simulink model "TV_comparison"  (R2022a)
settings: Solver=VariableStepAuto  StartTime=0.0  StopTime=140  RelTol=1e-3
values from neighbouring files (symbols this model uses):
  Battery_Voltage = 120    [RCVD.mat]
  CG_height = 0.6    [RCVD.mat]
  Cornering_Stiffness = 1000    [RCVD.mat]
  Gear_ratio = 6    [RCVD.mat]
  Mass = 250    [RCVD.mat]
  track_cumulative = tc.track_cumulative    [mlx_is_terrible.m]    (also in track.mat = [-1 0 1 0 0 -1 1 0 -1 1 -1 1 ... (560 elements, 140x4)])
  Wheel_Base = 1.8    [RCVD.mat]
  Wheel_Radius = 0.211    [RCVD.mat]
  Width = 1    [RCVD.mat]
libraries: SignalEditorBlockLib x4, autolibmappedmotor x2
settings Model: Creator=gautamd  LastModifiedBy=gautamd

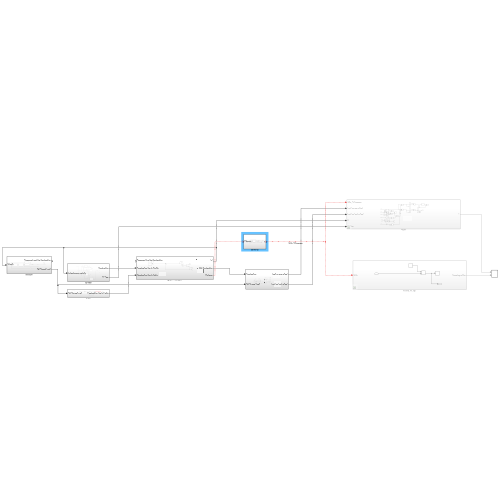
[thumbnail: Simulink's stored preview of the top-level diagram]
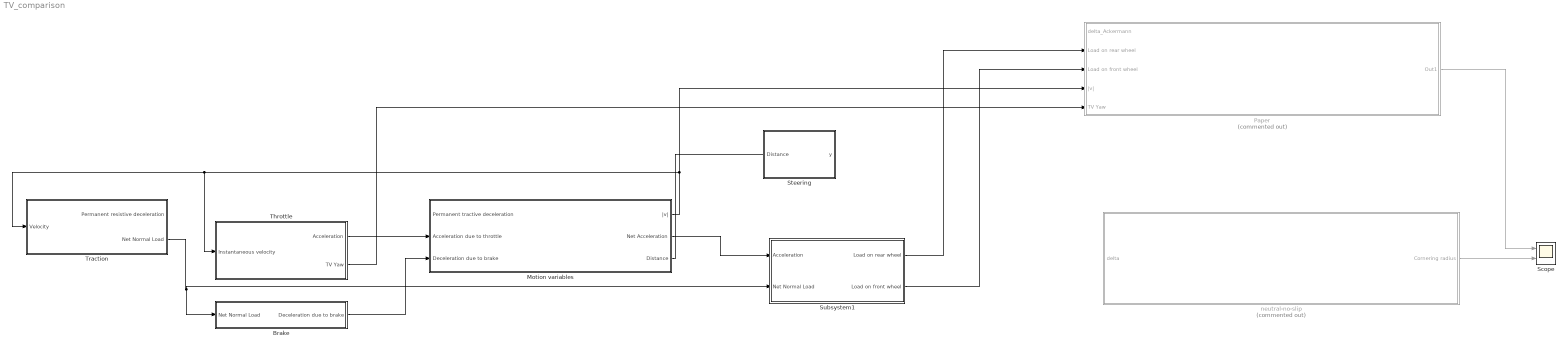
== system TV_comparison ==
  Brake : Subsystem
  Motion variables : Subsystem
  Paper : Subsystem  Commented=on
  Scope : Scope  NumInputPorts=2
  Steering : Subsystem
  Subsystem1 : Subsystem
  Throttle : Subsystem
  Traction : Subsystem
  neutral-no-slip : Subsystem  Commented=on
  wires:
  ? -> neutral-no-slip/1(delta), Paper/1(delta_Ackermann)  "delta_Ackermann"
  Subsystem1/1(Load on rear wheel) -> Paper/2(Load on rear wheel)
  Motion variables/2(Net Acceleration) -> Subsystem1/1(Acceleration)
  Subsystem1/2(Load on front wheel) -> Paper/3(Load on front wheel)
  Throttle/2(TV Yaw) -> Paper/5(TV Yaw)
  neutral-no-slip/1(Cornering radius) -> Scope/2
  Motion variables/1(|v|) -> Traction/1(Velocity), Throttle/1(Instantaneous velocity), Paper/4(|v|)
  Throttle/1(Acceleration) -> Motion variables/2(Acceleration due to throttle)
  Traction/2(Net Normal Load) -> Brake/1(Net Normal Load), Subsystem1/2(Net Normal Load)
  Paper/1(Out1) -> Scope/1
  Brake/1(Deceleration due to brake) -> Motion variables/3(Deceleration due to brake)
  Motion variables/3(Distance) -> ?

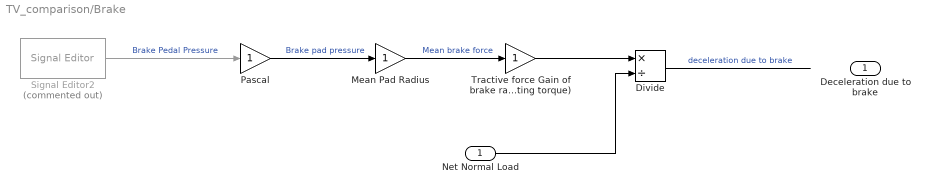
== system TV_comparison/Brake ==
  Net Normal Load : Inport
  Divide : Product  Inputs=*/
  Mean Pad Radius : Gain
  Pascal : Gain
  Signal Editor2 : SignalEditorBlockLib/Signal Editor  Commented=on  FileName=Brake_map.mat  ActiveScenario=Scenario  ActiveSignal=Signal 1  IsBus=off  OutputBusObjectStr=Bus: BusObject  SampleTime=0  Interpolate=off  ZeroCross=off  OutputAfterFinalValue=Setting to zero  Unit=inherit  PreserveSignalName=on
  Tractive force Gain of brake radius / wheel radius (equating torque) : Gain
  Deceleration due to brake : Outport
  wires:
  Signal Editor2/1 -> Pascal/1  "Brake Pedal Pressure"
  Pascal/1 -> Mean Pad Radius/1  "Brake pad pressure"
  Mean Pad Radius/1 -> Tractive force Gain of brake radius / wheel radius (equating torque)/1  "Mean brake force"
  Tractive force Gain of brake radius / wheel radius (equating torque)/1 -> Divide/1
  Divide/1 -> ?  "deceleration due to brake"
  Net Normal Load/1 -> Divide/2

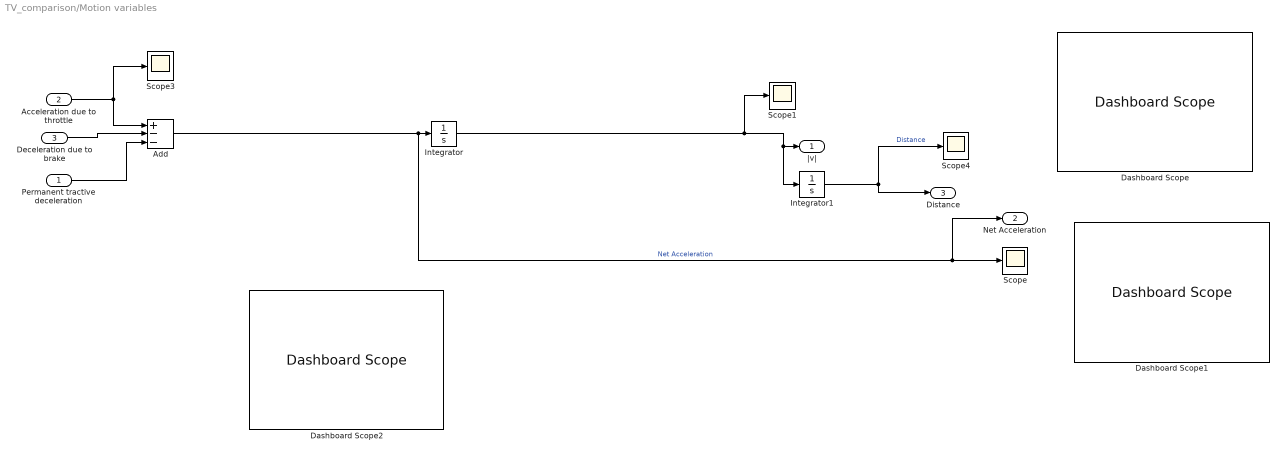
== system TV_comparison/Motion variables ==
  Permanent tractive deceleration : Inport
  Acceleration due to throttle : Inport  Port=2
  Deceleration due to brake : Inport  Port=3
  Add : Sum  Inputs=+--
  Dashboard Scope : DashboardScope
  Dashboard Scope1 : DashboardScope
  Dashboard Scope2 : DashboardScope
  Integrator : Integrator
  Integrator1 : Integrator
  Scope{,1,3..4} (4 alike) : Scope
  |v| : Outport
  Net Acceleration : Outport  Port=2
  Distance : Outport  Port=3
  wires:
  Integrator1/1 -> Scope4/1, Distance/1  "Distance"
  Add/1 -> Net Acceleration/1, Scope/1, Integrator/1  "Net Acceleration"
  Permanent tractive deceleration/1 -> Add/3
  Acceleration due to throttle/1 -> Add/1, Scope3/1
  Deceleration due to brake/1 -> Add/2
  Integrator/1 -> Scope1/1, Integrator1/1, |v|/1

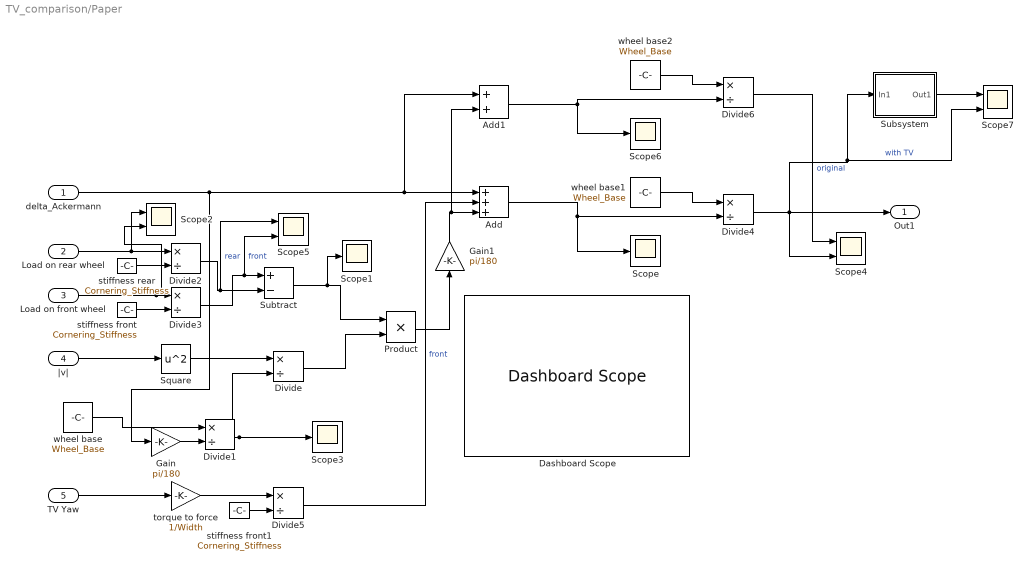
== system TV_comparison/Paper ==
  delta_Ackermann : Inport
  Load on rear wheel : Inport  Port=2
  Load on front wheel : Inport  Port=3
  |v| : Inport  Port=4
  TV Yaw : Inport  Port=5
  Add : Sum  Inputs=+++
  Add1 : Sum
  Dashboard Scope : DashboardScope
  Divide{,1..6} (7 alike) : Product  Inputs=*/
  Gain : Gain  Gain=pi/180
  Gain1 : Gain  Gain=pi/180
  Product : Product
  Scope{,1,3,6} (4 alike) : Scope
  Scope{2,4..5,7} (4 alike) : Scope  NumInputPorts=2
  Square : Math  Operator=square
  Subsystem : Subsystem
  Subtract : Sum  Inputs=+-
  stiffness front : Constant  Value=Cornering_Stiffness
  stiffness front1 : Constant  Value=Cornering_Stiffness
  stiffness rear : Constant  Value=Cornering_Stiffness
  torque to force : Gain  Gain=1/Width
  wheel base : Constant  Value=Wheel_Base
  wheel base1 : Constant  Value=Wheel_Base
  wheel base2 : Constant  Value=Wheel_Base
  Out1 : Outport
  wires:
  delta_Ackermann/1 -> Gain/1, Add1/1, Add/1
  |v|/1 -> Square/1
  Square/1 -> Divide/1
  wheel base/1 -> Divide1/1
  Divide1/1 -> Divide/2, Scope3/1
  Load on rear wheel/1 -> Scope2/1, Divide2/1
  Load on front wheel/1 -> Scope2/2, Divide3/1
  stiffness rear/1 -> Divide2/2
  stiffness front/1 -> Divide3/2
  Divide3/1 -> Scope5/2, Subtract/1  "front"
  Divide2/1 -> Subtract/2, Scope5/1  "rear"
  Subtract/1 -> Scope1/1, Product/1
  Divide/1 -> Product/2
  Product/1 -> Gain1/1
  Add/1 -> Divide4/2, Scope/1
  Gain/1 -> Divide1/2
  Divide4/1 -> Scope7/2, Subsystem/1(In1), Scope4/2, Out1/1  "with TV"
  wheel base1/1 -> Divide4/1
  Gain1/1 -> Add1/2, Add/3
  TV Yaw/1 -> torque to force/1
  torque to force/1 -> Divide5/1
  stiffness front1/1 -> Divide5/2
  Divide5/1 -> Add/2  "front"
  wheel base2/1 -> Divide6/1
  Add1/1 -> Divide6/2, Scope6/1
  Divide6/1 -> Scope4/1  "original"
  Subsystem/1(Out1) -> Scope7/1

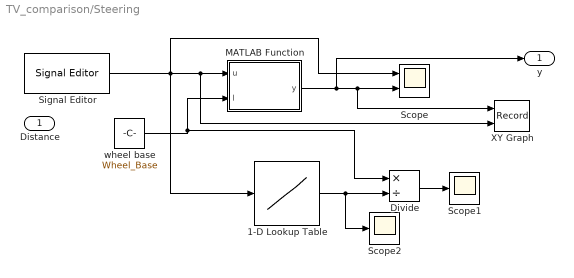
== system TV_comparison/Steering ==
  Distance : Inport
  1-D Lookup Table : Lookup_n-D  NumberOfTableDimensions=1  BreakpointsForDimension1=track_cumulative(:,4,:) - track_cumulative(:,2,:)  Table=track_cumulative(:,3,:).*track_cumulative(:,1,:)  InterpMethod=Flat  InternalRulePriority=Speed  RndMeth=Simplest
  Divide : Product  Inputs=*/
  MATLAB Function : MATLAB Function  TreatAsAtomicUnit=on
  Scope : Scope  NumInputPorts=2
  Scope1 : Scope
  Scope2 : Scope
  Signal Editor : SignalEditorBlockLib/Signal Editor  FileName=temp_distance_vs_time.mat  ActiveScenario=Scenario  ActiveSignal=Signal 1  IsBus=off  OutputBusObjectStr=Bus: BusObject  SampleTime=0  ZeroCross=off  OutputAfterFinalValue=Setting to zero  Unit=inherit  PreserveSignalName=on
  XY Graph : Record  FileSettingsInternal="{\"entries\":[{\"content\":{\"excelSettings\":{\"content\":{},\"type\":\"Streamout.ExcelSettings\"}},\"type\":\"Streamout.FileSettingStorage\",\"uuid\":\"\"}],\"packageUris\":[\"http:\\/\\/schema.mathworks.com\\/mf0\\/streamout_blocks\\/R2020a\"],\"version\":\"1.0\"}"  Layout=[1 1]  SignalsInternal="{\"entries\":[{\"content\":{\"signals\":[{\"content\":{\"blockPath\":[],\"channel\":[],\"dimensions\":[1],\"domain\":\"\",\"lineColor\":\"#a2142f\",\"plots\":[],\"port\":1,\"sid\":[\"\"],\"signalID\":2948,\"signalName\":\"MATLAB Function\"},\"type\":\"RecordBlkView.Signal\",\"uuid\":\"\"},{\"content\":{\"blockPath\":[],\"channel\":[],\"dimensions\":[1],\"domain\":\"\",\"lineColor\":\"#139fff\",\"plots\":[],\"port\":2,\"sid\":[\"\"],\"signalID\":2952,\"signalName\":\"Signal Editor\"},\"type\":\"RecordBlkView.Signal\",\"uuid\":\"\"}]},\"type\":\"RecordBlkView.InputSignals\",\"uuid\":\"\"}],\"packageUris\":[\"http:\\/\\/schema.mathworks.com\\/mf0\\/streamout_blocks\\/R2020a\"],\"version\":\"1.0\"}"  VisualizationBindings="{\"xyplotplugin\":{\"info\":[{\"series\":[],\"subplotID\":1}]}}"  CompatibilityTag=XY
  wheel base : Constant  Value=Wheel_Base
  y : Outport
  wires:
  Signal Editor/1 -> 1-D Lookup Table/1, Scope/1, XY Graph/2, MATLAB Function/1(u)
  wheel base/1 -> Divide/1, MATLAB Function/2(l)
  MATLAB Function/1(y) -> y/1, XY Graph/1, Scope/2
  1-D Lookup Table/1 -> Scope2/1, Divide/2
  Divide/1 -> Scope1/1

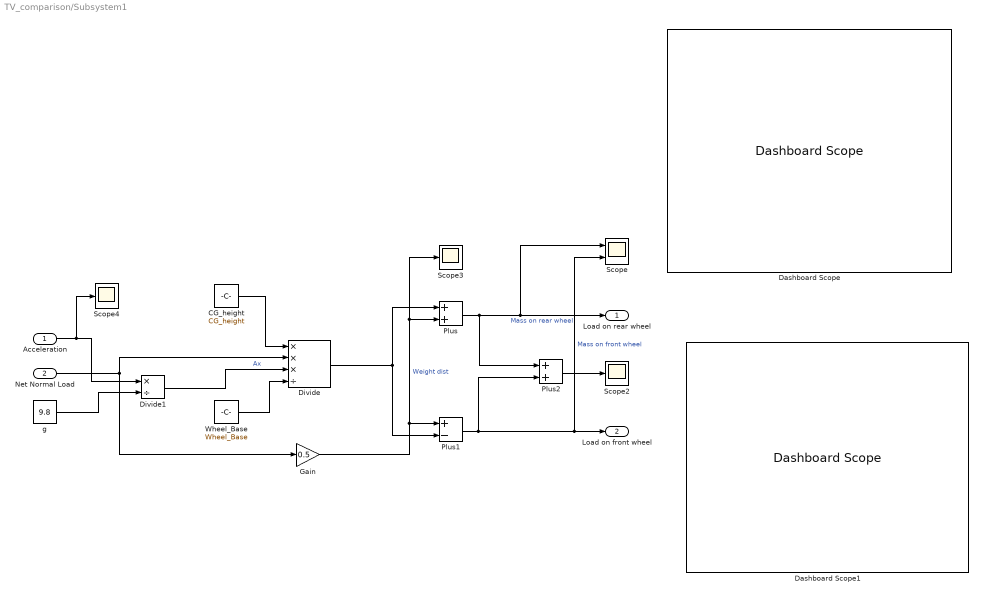
== system TV_comparison/Subsystem1 ==
  Acceleration : Inport
  Net Normal Load : Inport  Port=2
  CG_height : Constant  Value=CG_height
  Dashboard Scope : DashboardScope
  Dashboard Scope1 : DashboardScope
  Divide : Product  Inputs=***/
  Divide1 : Product  Inputs=*/
  Gain : Gain  Gain=0.5
  Plus : Sum
  Plus1 : Sum  Inputs=+-
  Plus2 : Sum
  Scope : Scope  NumInputPorts=2
  Scope2 : Scope
  Scope3 : Scope
  Scope4 : Scope
  Wheel_Base : Constant  Value=Wheel_Base
  g : Constant  Value=9.8
  Load on rear wheel : Outport
  Load on front wheel : Outport  Port=2
  wires:
  g/1 -> Divide1/2
  Divide/1 -> Plus1/2, Plus/1
  Acceleration/1 -> Scope4/1, Divide1/1
  Gain/1 -> Scope3/1, Plus/2, Plus1/1  "Weight dist"
  CG_height/1 -> Divide/1
  Wheel_Base/1 -> Divide/4
  Divide1/1 -> Divide/3  "Ax"
  Plus/1 -> Scope/1, Load on rear wheel/1, Plus2/1  "Mass on rear wheel"
  Plus1/1 -> Scope/2, Load on front wheel/1, Plus2/2  "Mass on front wheel"
  Net Normal Load/1 -> Divide/2, Gain/1
  Plus2/1 -> Scope2/1

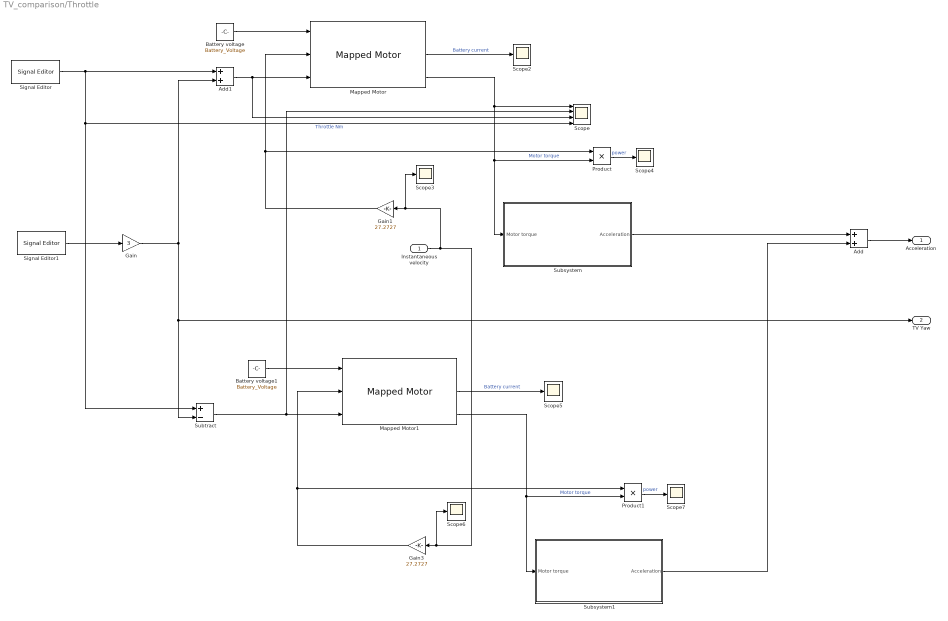
== system TV_comparison/Throttle ==
  Instantaneous velocity : Inport
  Add : Sum
  Add1 : Sum
  Battery voltage : Constant  Value=Battery_Voltage
  Battery voltage1 : Constant  Value=Battery_Voltage
  Gain : Gain  Gain=3
  Gain1 : Gain  Gain=27.2727
  Gain3 : Gain  Gain=27.2727
  Mapped Motor : autolibmappedmotor/Mapped Motor  port_config=Speed  param_by=Maximum torque and power  w_t=[ 0 375 750 800 ]  T_t=[0.09 0.08 0.07 0]  torque_max=29  power_max=Max_Power  Tc=0.1  param_loss=Single efficiency measurement  eff=93  w_eff=600  T_eff=29  Piron=0  Pbase=0  w_eff_bp=[-8000 -4000 0 4000 8000]  T_eff_bp=[0 0.03 0.06 0.09]  Temp_eff_bp=[233.15 293.15 373.15]  losses_table=[1.49 1.67 2.21 3.10; 0.42 0.69 1.14 2.03; 0.06 0.24 0.78 1.68; 0.42 0.69 1.14 2.03; 1.49 1.67 2.21 3.10]  losses_table_3d=cat(3,1.05*[1.49 1.67 2.21 3.10; 0.42 0.69 1.14 2.03; 0.06 0.24 0.78 1.68; 0.42 0.69 1.14 2.03; 1.49 1.67 2.21 3.10],[1.49 1.67 2.21 3.10; 0.42 0.69 1.14 2.03; 0.06 0.24 0.78 1.68; 0.42 0.69 1.14 2.03; 1.49 1.67 2.21 3.10],1.03*[1.49 1.67 2.21 3.10; 0.42 0.69 1.14 2.03; 0.06 0.24 0.78 1.68; 0.42 0.69 1.14 2.03; 1.49 1.67 2.21 3.10])  efficiency_table=[95 95 95 95; 95 95 95 95; 95 95 95 95; 95 95 95 95; 95 95 95 95]  efficiency_table_3d=cat(3,90*ones(5,4),95*ones(5,4),92*ones(5,4))  J=0.021  b=1e-5  omega_o=0  T_t_extended=[0 0.07 0.08 0.09 0.08 0.07 0]  w_t_extended=[-800 -750 -375 0 375 750 800]  KLossIron=0  KLossCopper=1.5573  x_w_eff_vec=[-8000 -4000 0 4000 8000]  x_T_eff_vec=[-0.09 -0.06 -0.03 0 0.03 0.06 0.09]  x_tmp_eff_vec=[233.15 293.15 373.15]  x_losses_mat=[3.1 2.21 1.67 1.49 1.67 2.21 3.1;2.03 1.14 0.69 0.42 0.69 1.14 2.03;1.68 0.78 0.24 0.06 0.24 0.78 1.68;2.03 1.14 0.69 0.42 0.69 1.14 2.03;3.1 2.21 1.67 1.49 1.67 2.21 3.1]  x_losses_mat_3d=cat(3,[3.255 2.3205 1.7535 1.5645 1.7535 2.3205 3.255;2.1315 1.197 0.7245 0.441 0.7245 1.197 2.1315;1.764 0.819 0.252 0.063 0.252 0.819 1.764;2.1315 1.197 0.7245 0.441 0.7245 1.197 2.1315;3.255 2.3205 1.7535 1.5645 1.7535 2.3205 3.255],[3.1 2.21 1.67 1.49 1.67 2.21 3.1;2.03 1.14 0.69 0.42 0.69 1.14 2.03;1.68 0.78 0.24 0.06 0.24 0.78 1.68;2.03 1.14 0.69 0.42 0.69 1.14 2.03;3.1 2.21 1.67 1.49 1.67 2.21 3.1],[3.193 2.2763 1.7201 1.5347 1.7201 2.2763 3.193;2.0909 1.1742 0.7107 0.4326 0.7107 1.1742 2.0909;1.7304 0.8034 0.2472 0.0618 0.2472 0.8034 1.7304;2.0909 1.1742 0.7107 0.4326 0.7107 1.1742 2.0909;3.193 2.2763 1.7201 1.5347 1.7201 2.2763 3.193])  CalLossMapData={}  CalLossWithTempMapData={}  aMode=2  RefBlkName='autolibmappedmotor/Mapped Motor'
      settings: SourceProductBaseCode=PW,DR,MT,VE
  Mapped Motor1 : autolibmappedmotor/Mapped Motor  port_config=Speed  param_by=Maximum torque and power  w_t=[ 0 375 750 800 ]  T_t=[0.09 0.08 0.07 0]  torque_max=29  power_max=Max_Power  Tc=0.1  param_loss=Single efficiency measurement  eff=93  w_eff=600  T_eff=29  Piron=0  Pbase=0  w_eff_bp=[-8000 -4000 0 4000 8000]  T_eff_bp=[0 0.03 0.06 0.09]  Temp_eff_bp=[233.15 293.15 373.15]  losses_table=[1.49 1.67 2.21 3.10; 0.42 0.69 1.14 2.03; 0.06 0.24 0.78 1.68; 0.42 0.69 1.14 2.03; 1.49 1.67 2.21 3.10]  losses_table_3d=cat(3,1.05*[1.49 1.67 2.21 3.10; 0.42 0.69 1.14 2.03; 0.06 0.24 0.78 1.68; 0.42 0.69 1.14 2.03; 1.49 1.67 2.21 3.10],[1.49 1.67 2.21 3.10; 0.42 0.69 1.14 2.03; 0.06 0.24 0.78 1.68; 0.42 0.69 1.14 2.03; 1.49 1.67 2.21 3.10],1.03*[1.49 1.67 2.21 3.10; 0.42 0.69 1.14 2.03; 0.06 0.24 0.78 1.68; 0.42 0.69 1.14 2.03; 1.49 1.67 2.21 3.10])  efficiency_table=[95 95 95 95; 95 95 95 95; 95 95 95 95; 95 95 95 95; 95 95 95 95]  efficiency_table_3d=cat(3,90*ones(5,4),95*ones(5,4),92*ones(5,4))  J=0.021  b=1e-5  omega_o=0  T_t_extended=[0 0.07 0.08 0.09 0.08 0.07 0]  w_t_extended=[-800 -750 -375 0 375 750 800]  KLossIron=0  KLossCopper=1.5573  x_w_eff_vec=[-8000 -4000 0 4000 8000]  x_T_eff_vec=[-0.09 -0.06 -0.03 0 0.03 0.06 0.09]  x_tmp_eff_vec=[233.15 293.15 373.15]  x_losses_mat=[3.1 2.21 1.67 1.49 1.67 2.21 3.1;2.03 1.14 0.69 0.42 0.69 1.14 2.03;1.68 0.78 0.24 0.06 0.24 0.78 1.68;2.03 1.14 0.69 0.42 0.69 1.14 2.03;3.1 2.21 1.67 1.49 1.67 2.21 3.1]  x_losses_mat_3d=cat(3,[3.255 2.3205 1.7535 1.5645 1.7535 2.3205 3.255;2.1315 1.197 0.7245 0.441 0.7245 1.197 2.1315;1.764 0.819 0.252 0.063 0.252 0.819 1.764;2.1315 1.197 0.7245 0.441 0.7245 1.197 2.1315;3.255 2.3205 1.7535 1.5645 1.7535 2.3205 3.255],[3.1 2.21 1.67 1.49 1.67 2.21 3.1;2.03 1.14 0.69 0.42 0.69 1.14 2.03;1.68 0.78 0.24 0.06 0.24 0.78 1.68;2.03 1.14 0.69 0.42 0.69 1.14 2.03;3.1 2.21 1.67 1.49 1.67 2.21 3.1],[3.193 2.2763 1.7201 1.5347 1.7201 2.2763 3.193;2.0909 1.1742 0.7107 0.4326 0.7107 1.1742 2.0909;1.7304 0.8034 0.2472 0.0618 0.2472 0.8034 1.7304;2.0909 1.1742 0.7107 0.4326 0.7107 1.1742 2.0909;3.193 2.2763 1.7201 1.5347 1.7201 2.2763 3.193])  CalLossMapData={}  CalLossWithTempMapData={}  aMode=2  RefBlkName='autolibmappedmotor/Mapped Motor'
      settings: SourceProductBaseCode=PW,DR,MT,VE
  Product : Product
  Product1 : Product
  Scope : Scope  NumInputPorts=4
  Scope{2..7} (6 alike) : Scope
  Signal Editor : SignalEditorBlockLib/Signal Editor  FileName=Throttle_map.mat  ActiveScenario=Scenario  ActiveSignal=Signal 1  IsBus=off  OutputBusObjectStr=Bus: BusObject  SampleTime=0  Interpolate=off  ZeroCross=off  OutputAfterFinalValue=Setting to zero  Unit=inherit  PreserveSignalName=on
  Signal Editor1 : SignalEditorBlockLib/Signal Editor  FileName=Torque vectoring input.mat  ActiveScenario=Scenario  ActiveSignal=Signal 1  IsBus=off  OutputBusObjectStr=Bus: BusObject  SampleTime=0  Interpolate=off  ZeroCross=off  OutputAfterFinalValue=Setting to zero  Unit=inherit  PreserveSignalName=on
  Subsystem : Subsystem
  Subsystem1 : Subsystem
  Subtract : Sum  Inputs=+-
  Acceleration : Outport
  TV Yaw : Outport  Port=2
  wires:
  Battery voltage/1 -> Mapped Motor/1
  Signal Editor/1 -> Scope/4, Subtract/1, Add1/1  "Throttle Nm"
  Mapped Motor/2 -> Scope2/1  "Battery current"
  Mapped Motor/3 -> Product/2, Subsystem/1(Motor torque), Scope/1  "Motor torque"
  Gain1/1 -> Product/1, Mapped Motor/2
  Product/1 -> Scope4/1  "power"
  Subsystem1/1(Acceleration) -> Add/2
  Product1/1 -> Scope7/1  "power"
  Mapped Motor1/2 -> Scope5/1  "Battery current"
  Mapped Motor1/3 -> Product1/2, Subsystem1/1(Motor torque)  "Motor torque"
  Instantaneous velocity/1 -> Scope6/1, Gain3/1, Scope3/1, Gain1/1
  Gain3/1 -> Product1/1, Mapped Motor1/2
  Battery voltage1/1 -> Mapped Motor1/1
  Add/1 -> Acceleration/1
  Subsystem/1(Acceleration) -> Add/1
  Signal Editor1/1 -> Gain/1
  Add1/1 -> Scope/3, Mapped Motor/3
  Subtract/1 -> Scope/2, Mapped Motor1/3
  Gain/1 -> Add1/2, TV Yaw/1, Subtract/2

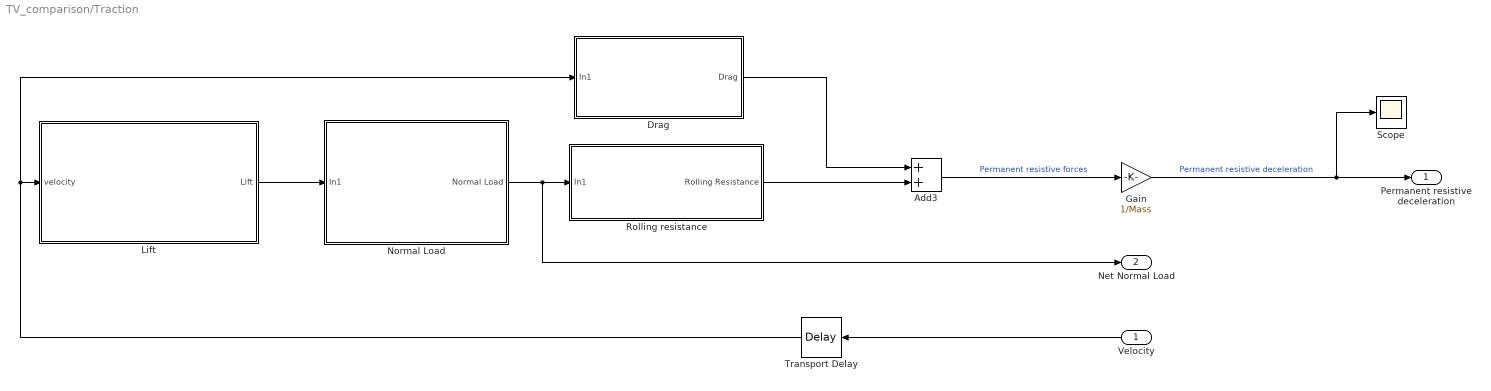
== system TV_comparison/Traction ==
  Velocity : Inport
  Add3 : Sum
  Drag : Subsystem
  Gain : Gain  Gain=1/Mass
  Lift : Subsystem
  Normal Load : Subsystem
  Rolling resistance : Subsystem
  Scope : Scope
  Transport Delay : TransportDelay  DelayTime=0.1
  Permanent resistive deceleration : Outport
  Net Normal Load : Outport  Port=2
  wires:
  Velocity/1 -> Transport Delay/1
  Lift/1(Lift) -> Normal Load/1(In1)
  Rolling resistance/1(Rolling Resistance) -> Add3/2
  Transport Delay/1 -> Drag/1(In1), Lift/1(velocity)
  Normal Load/1(Normal Load) -> Net Normal Load/1, Rolling resistance/1(In1)
  Drag/1(Drag) -> Add3/1
  Gain/1 -> Scope/1, Permanent resistive deceleration/1  "Permanent resistive deceleration"
  Add3/1 -> Gain/1  "Permanent resistive forces"

== system TV_comparison/neutral-no-slip ==
  delta : Inport
  Divide1 : Product  Inputs=*/
  Scope7 : Scope
  Wheel Base : Constant  Value=Wheel_Base
  Cornering radius : Outport
  wires:
  Wheel Base/1 -> Divide1/1
  Divide1/1 -> Cornering radius/1, Scope7/1  "R"
  delta/1 -> Divide1/2  "net delta"

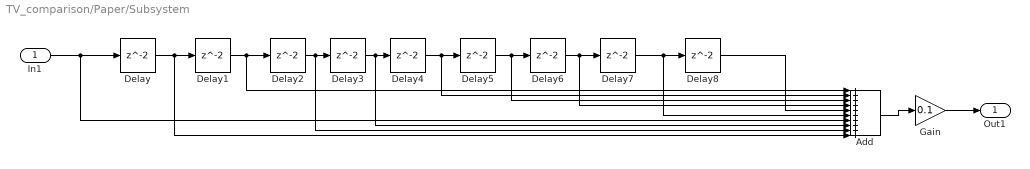
== system TV_comparison/Paper/Subsystem ==
  In1 : Inport
  Add : Sum  Inputs=++++++++++
  Delay : Delay  SampleTime=0.01
  Delay{1..8} (8 alike) : Delay
  Gain : Gain  Gain=0.1
  Out1 : Outport
  wires:
  Delay/1 -> Add/10, Delay1/1
  In1/1 -> Add/7, Delay/1
  Delay1/1 -> Add/1, Delay2/1
  Delay2/1 -> Add/9, Delay3/1
  Delay3/1 -> Add/8, Delay4/1
  Delay4/1 -> Add/2, Delay5/1
  Delay5/1 -> Add/3, Delay6/1
  Delay6/1 -> Add/4, Delay7/1
  Add/1 -> Gain/1
  Delay7/1 -> Delay8/1, Add/6
  Gain/1 -> Out1/1
  Delay8/1 -> Add/5

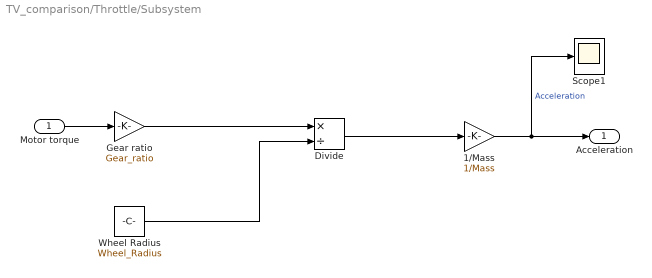
== system TV_comparison/Throttle/Subsystem ==
  Motor torque : Inport
  1/Mass : Gain  Gain=1/Mass
  Divide : Product  Inputs=*/
  Gear ratio : Gain  Gain=Gear_ratio
  Scope1 : Scope
  Wheel Radius : Constant  Value=Wheel_Radius
  Acceleration : Outport
  wires:
  Divide/1 -> 1/Mass/1
  Gear ratio/1 -> Divide/1
  Wheel Radius/1 -> Divide/2
  1/Mass/1 -> Acceleration/1, Scope1/1  "Acceleration"
  Motor torque/1 -> Gear ratio/1

== system TV_comparison/Throttle/Subsystem1 ==
  Motor torque : Inport
  1/Mass : Gain  Gain=1/Mass
  Divide : Product  Inputs=*/
  Gear ratio : Gain  Gain=Gear_ratio
  Scope1 : Scope
  Wheel Radius : Constant  Value=Wheel_Radius
  Acceleration : Outport
  wires:
  Divide/1 -> 1/Mass/1
  Gear ratio/1 -> Divide/1
  Wheel Radius/1 -> Divide/2
  1/Mass/1 -> Acceleration/1, Scope1/1  "Acceleration"
  Motor torque/1 -> Gear ratio/1

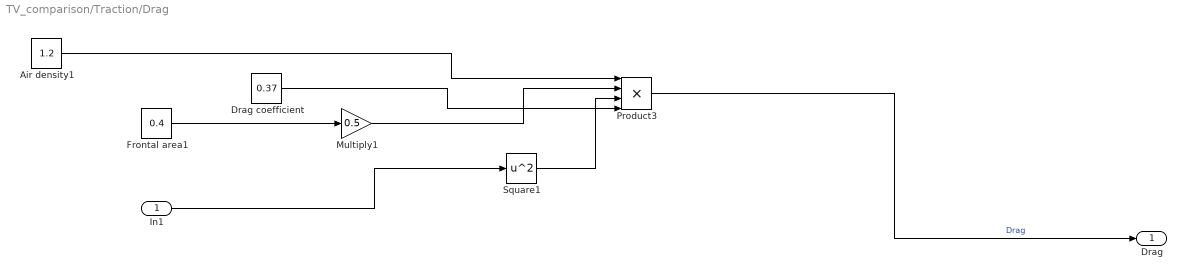
== system TV_comparison/Traction/Drag ==
  In1 : Inport
  Air density1 : Constant  Value=1.2
  Drag coefficient : Constant  Value=0.37
  Frontal area1 : Constant  Value=0.4
  Multiply1 : Gain  Gain=0.5
  Product3 : Product  Inputs=4
  Square1 : Math  Operator=square
  Drag : Outport
  wires:
  Multiply1/1 -> Product3/2
  Square1/1 -> Product3/3
  In1/1 -> Square1/1
  Air density1/1 -> Product3/1
  Frontal area1/1 -> Multiply1/1
  Drag coefficient/1 -> Product3/4
  Product3/1 -> Drag/1  "Drag"

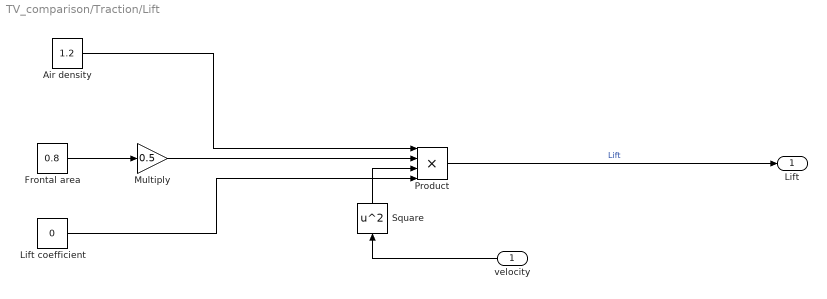
== system TV_comparison/Traction/Lift ==
  velocity : Inport
  Air density : Constant  Value=1.2
  Frontal area : Constant  Value=0.8
  Lift coefficient : Constant  Value=0
  Multiply : Gain  Gain=0.5
  Product : Product  Inputs=4
  Square : Math  Operator=square
  Lift : Outport
  wires:
  Frontal area/1 -> Multiply/1
  Multiply/1 -> Product/2
  Lift coefficient/1 -> Product/4
  Air density/1 -> Product/1
  Square/1 -> Product/3
  velocity/1 -> Square/1
  Product/1 -> Lift/1  "Lift"

== system TV_comparison/Traction/Normal Load ==
  In1 : Inport
  Add1 : Sum  Inputs=+-
  Mass : Constant  Value=Mass
  Product1 : Product
  g : Constant  Value=9.8
  Normal Load : Outport
  wires:
  g/1 -> Product1/1
  Product1/1 -> Add1/1  "Car weight"
  Mass/1 -> Product1/2
  Add1/1 -> Normal Load/1  "Normal Load"
  In1/1 -> Add1/2

== system TV_comparison/Traction/Rolling resistance ==
  In1 : Inport
  Product5 : Product
  Rolling resistance coefficient : Constant  Value=0
  Rolling Resistance : Outport
  wires:
  Rolling resistance coefficient/1 -> Product5/1
  Product5/1 -> Rolling Resistance/1  "Rolling Resistance"
  In1/1 -> Product5/2

== matlab function TV_comparison/Steering/MATLAB Function ==
  data: u input; y output; l input
function y = fcn(u, l)

if u < 2.91
	y = l/4.86000000000000;
elseif u < 13.9
	y = 0;
elseif u < 17.45
	y = l/4.86000000000000;
elseif u < 40.81
	y = 0;
elseif u < 52.39
	y = 0;
elseif u < 60.93
	y = l/5.84000000000000;
elseif u < 64.55
	y = l/2.92000000000000;
elseif u < 95.99
	y = 0;
elseif u < 98.83999999999999
	y = l/4;
elseif u < 105.72999999999999
	y = l/3.75000000000000;
elseif u < 109.07
	y = l/1.52000000000000;
elseif u < 113.69
	y = l/2.10000000000000;
elseif u < 118.16
	y = l/2.04000000000000;
elseif u < 122.44
	y = l/1.95000000000000;
elseif u < 126.89999999999999
	y = l/2.03000000000000;
elseif u < 130.89
	y = l/1.82000000000000;
elseif u < 135.04
	y = l/1.89000000000000;
elseif u < 139.32999999999998
	y = l/1.95000000000000;
elseif u < 142.35999999999999
	y = l/2.07000000000000;
elseif u < 147.32
	y = l/15.3200000000000;
elseif u < 162.76
	y = 0;
elseif u < 170.73999999999998
	y = l/8.53000000000000;
elseif u < 173.68999999999997
	y = l/1.80000000000000;
elseif u < 181.83999999999997
	y = 0;
elseif u < 187.93999999999997
	y = l/3.82000000000000;
elseif u < 193.25999999999996
	y = 0;
elseif u < 201.81999999999996
	y = l/4.69000000000000;
elseif u < 205.82999999999996
	y = 0;
elseif u < 214.24999999999994
	y = l/4.14000000000000;
elseif u < 224.34999999999994
	y = l/7.54000000000000;
elseif u < 224.44999999999993
	y = 0;
elseif u < 226.03999999999994
	y = l/3.94000000000000;
elseif u < 226.13999999999993
	y = 0;
elseif u < 228.33999999999992
	y = l/2.92000000000000;
elseif u < 231.26999999999992
	y = 0;
elseif u < 235.33999999999992
	y = l/2.34000000000000;
elseif u < 237.7299999999999
	y = l/6.94000000000000;
elseif u < 313.1199999999999
	y = 0;
elseif u < 321.1299999999999
	y = l/12.3300000000000;
elseif u < 328.46999999999986
	y = l/5.73000000000000;
elseif u < 332.14999999999986
	y = l/2.87000000000000;
elseif u < 335.6399999999999
	y = l/2.73000000000000;
elseif u < 339.9899999999999
	y = l/3.40000000000000;
elseif u < 343.3099999999999
	y = l/2.59000000000000;
elseif u < 347.08999999999986
	y = l/2.95000000000000;
elseif u < 350.36999999999983
	y = l/2.56000000000000;
elseif u < 352.99999999999983
	y = l/3.30000000000000;
elseif u < 358.46999999999986
	y = l/58.5400000000000;
elseif u < 393.21999999999986
	y = 0;
elseif u < 405.58999999999986
	y = l/13.5700000000000;
elseif u < 408.4999999999999
	y = l/2.92000000000000;
elseif u < 450.3199999999999
	y = 0;
elseif u < 462.46999999999986
	y = l/10.3900000000000;
elseif u < 462.5699999999999
	y = 0;
elseif u < 521.4699999999999
	y = l/81.5500000000000;
elseif u < 521.5699999999999
	y = 0;
elseif u < 530.1099999999999
	y = l/14.7500000000000;
elseif u < 530.2099999999999
	y = 0;
elseif u < 557.1999999999999
	y = l/15.6300000000000;
elseif u < 572.5099999999999
	y = l/15.1600000000000;
elseif u < 576.3699999999999
	y = 0;
elseif u < 591.31
	y = 0;
elseif u < 606.01
	y = l/59.0400000000000;
elseif u < 606.11
	y = 0;
elseif u < 613.1800000000001
	y = l/8.50000000000000;
elseif u < 626.82
	y = l/8.68000000000000;
elseif u < 639.35
	y = l/7.98000000000000;
elseif u < 651.39
	y = l/7.66000000000000;
elseif u < 663.55
	y = l/10.2200000000000;
elseif u < 674.5699999999999
	y = l/26.8600000000000;
elseif u < 706.31
	y = 0;
elseif u < 714.9599999999999
	y = l/15.1800000000000;
elseif u < 735.3
	y = l/13.4200000000000;
elseif u < 742.51
	y = 0;
elseif u < 766.63
	y = l/16.4300000000000;
elseif u < 767.74
	y = l/2.92000000000000;
elseif u < 767.84
	y = 0;
elseif u < 773.21
	y = l/5.99000000000000;
elseif u < 788.14
	y = l/6.38000000000000;
elseif u < 801.72
	y = l/4.48000000000000;
elseif u < 814.9200000000001
	y = l/4.10000000000000;
elseif u < 828.6700000000001
	y = l/4.78000000000000;
elseif u < 839.84
	y = l/5.27000000000000;
elseif u < 841.0600000000001
	y = l/4.86000000000000;
elseif u < 844.4200000000001
	y = 0;
elseif u < 848.4300000000001
	y = l/4.86000000000000;
elseif u < 859.86
	y = 0;
elseif u < 860.66
	y = l/4.86000000000000;
elseif u < 883.5699999999999
	y = l/118.360000000000;
elseif u < 883.67
	y = 0;
elseif u < 900.64
	y = l/24.7400000000000;
elseif u < 916.4499999999999
	y = l/84.6500000000000;
elseif u < 939.2599999999999
	y = 0;
elseif u < 968.1399999999999
	y = l/66.1800000000000;
elseif u < 982.3599999999999
	y = 0;
elseif u < 1002.4599999999999
	y = 0;
elseif u < 1010.2699999999999
	y = l/31.5700000000000;
elseif u < 1017.4599999999999
	y = l/8.94000000000000;
elseif u < 1026.0
	y = l/7.78000000000000;
elseif u < 1034.7
	y = l/7.93000000000000;
elseif u < 1043.53
	y = l/8.05000000000000;
elseif u < 1055.35
	y = l/14.5100000000000;
elseif u < 1063.1399999999999
	y = l/69.3700000000000;
elseif u < 1063.2399999999998
	y = 0;
elseif u < 1075.8899999999999
	y = l/15.6000000000000;
elseif u < 1086.8799999999999
	y = 0;
elseif u < 1089.09
	y = l/4.86000000000000;
elseif u < 1102.82
	y = 0;
elseif u < 1104.36
	y = l/4.86000000000000;
elseif u < 1110.9199999999998
	y = 0;
elseif u < 1124.4599999999998
	y = l/4.31000000000000;
elseif u < 1131.2599999999998
	y = 0;
elseif u < 1134.4399999999998
	y = l/2.92000000000000;
elseif u < 1134.5399999999997
	y = 0;
elseif u < 1150.7199999999998
	y = l/11.4200000000000;
elseif u < 1162.4399999999998
	y = l/12.0700000000000;
elseif u < 1174.7499999999998
	y = 0;
elseif u < 1177.4799999999998
	y = l/4.86000000000000;
elseif u < 1197.2199999999998
	y = l/14.1800000000000;
elseif u < 1199.6399999999999
	y = l/2.92000000000000;
elseif u < 1206.34
	y = 0;
elseif u < 1212.1599999999999
	y = l/6.72000000000000;
elseif u < 1212.2599999999998
	y = 0;
elseif u < 1226.0399999999997
	y = l/10.4800000000000;
elseif u < 1241.0399999999997
	y = l/5.46000000000000;
elseif u < 1241.1399999999996
	y = 0;
elseif u < 1244.9599999999996
	y = l/4.34000000000000;
elseif u < 1245.0599999999995
	y = 0;
elseif u < 1256.7699999999995
	y = l/12.9200000000000;
elseif u < 1272.6199999999994
	y = l/9.09000000000000;
elseif u < 1278.9199999999994
	y = 0;
elseif u < 1282.4299999999994
	y = l/2.92000000000000;
elseif u < 1300.1499999999994
	y = 0;
elseif u < 1314.1399999999994
	y = l/8.91000000000000;
elseif u < 1318.6499999999994
	y = l/2.92000000000000;
elseif u < 1327.8799999999994
	y = 0;
elseif u < 1334.8799999999994
	y = l/5.82000000000000;
elseif u < 1337.5199999999995
	y = l/2.92000000000000;
elseif u < 1376.2399999999996
	y = 0;
else
    y = 0;
end
